simulink model "lista1_8"  (R2020a)
settings: Solver=FixedStepAuto  StartTime=0.0  StopTime=50  FixedStep=0.001  RelTol=1e-3
settings Model: Creator=bruno  LastModifiedBy=bruno

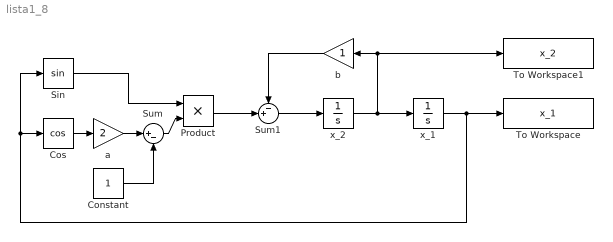
== system lista1_8 ==
  Constant : Constant
  Cos : Trigonometry  Operator=cos
  Product : Product
  Sin : Trigonometry
  Sum : Sum  Inputs=|+-
  Sum1 : Sum  Inputs=-+|
  To Workspace : ToWorkspace  VariableName=x_1  SaveFormat=Timeseries  SampleTime=-1
  To Workspace1 : ToWorkspace  VariableName=x_2  SaveFormat=Timeseries  SampleTime=-1
  a : Gain  Gain=2
  b : Gain
  x_1 : Integrator  InitialCondition=pi - 0.001
  x_2 : Integrator
  wires:
  x_2/1 -> x_1/1, To Workspace1/1, b/1
  x_1/1 -> To Workspace/1, Cos/1, Sin/1
  Cos/1 -> a/1
  a/1 -> Sum/1
  Constant/1 -> Sum/2
  Sum/1 -> Product/2
  Sin/1 -> Product/1
  Product/1 -> Sum1/2
  Sum1/1 -> x_2/1
  b/1 -> Sum1/1
